simulink model "model_ref_q6"  (R2020b)
settings: Solver=VariableStepAuto  StartTime=0.0  StopTime=10.0  RelTol=1e-3
settings Model: Creator=sneha  LastModifiedBy=sneha
settings DataIOCC: SaveOutput=off  SaveTime=off

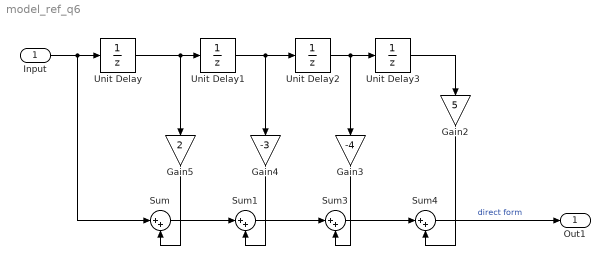
== system model_ref_q6 ==
  Input : Inport  OutDataTypeStr=double  PortDimensions=1  SampleTime=[0,1]
  Gain2 : Gain  Gain=5
  Gain3 : Gain  Gain=-4
  Gain4 : Gain  Gain=-3
  Gain5 : Gain  Gain=2
  Sum{,1,3..4} (4 alike) : Sum  Inputs=|++
  Unit Delay{,1..3} (4 alike) : UnitDelay  SampleTime=-1  HasFrameUpgradeWarning=on
  Out1 : Outport  OutDataTypeStr=double  PortDimensions=1  SampleTime=[0,1]
  wires:
  Sum/1 -> Sum1/1
  Unit Delay/1 -> Unit Delay1/1, Gain5/1
  Sum3/1 -> Sum4/1
  Input/1 -> Unit Delay/1, Sum/1
  Gain5/1 -> Sum/2
  Gain4/1 -> Sum1/2
  Gain3/1 -> Sum3/2
  Sum4/1 -> Out1/1  "direct form"
  Unit Delay2/1 -> Unit Delay3/1, Gain3/1
  Gain2/1 -> Sum4/2
  Unit Delay1/1 -> Gain4/1, Unit Delay2/1
  Sum1/1 -> Sum3/1
  Unit Delay3/1 -> Gain2/1
